simulink model "sudarshan_1"  (R2022b)
settings: Solver=ode4  StartTime=0.0  StopTime=5  FixedStep=0.0001  RelTol=1e-3
settings Model: Creator=year2  LastModifiedBy=year2

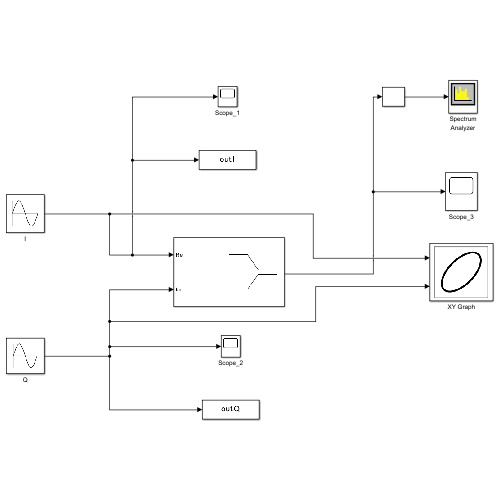
[thumbnail: Simulink's stored preview of the top-level diagram]
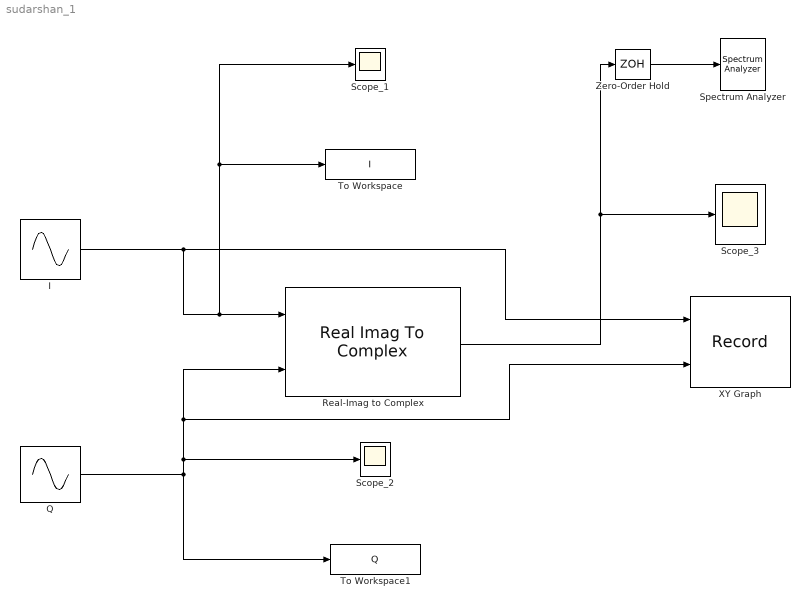
== system sudarshan_1 ==
  I : Sin  Frequency=100  Phase=pi/2  SampleTime=0
  Q : Sin  Frequency=100  SampleTime=0
  Real-Imag to Complex : RealImagToComplex
  Scope_1 : Scope
  Scope_2 : Scope
  Scope_3 : Scope
  Spectrum Analyzer : SpectrumAnalyzer
  To Workspace : ToWorkspace  VariableName=I  SaveFormat=Timeseries  SampleTime=-1
  To Workspace1 : ToWorkspace  VariableName=Q  SaveFormat=Timeseries  SampleTime=-1
  XY Graph : Record  FileSettingsInternal="{\"entries\":[{\"content\":{\"excelSettings\":{\"content\":{},\"type\":\"Streamout.ExcelSettings\"}},\"type\":\"Streamout.FileSettingStorage\",\"uuid\":\"9869a838-1e5d-41e2-a3ef-ea152b2475d8\"}],\"packageUris\":[\"http://schema.mathworks.com/mf0/streamout_blocks/R2020a\"],\"version\":\"1.0\"}"  Layout=[1 1]  SignalsInternal="{\"entries\":[{\"content\":{\"signals\":[{\"content\":{\"blockPath\":[\"sudarshan_1/XY Graph\"],\"channel\":[],\"dimensions\":[1],\"domain\":\"sudarshan_1/XY Graph\",\"lineColor\":\"#a2142f\",\"plots\":[1],\"port\":1,\"sid\":[\"\"],\"signalID\":933,\"signalName\":\"I\"},\"type\":\"RecordBlkView.Signal\",\"uuid\":\"0f210d62-b191-4474-a9fa-690a825850b4\"},{\"content\":{\"blockPath\":[\"sudarshan_1/XY Graph\"],\"channel\":[],\"dimensions\":[1],\"domain\":\"sudarshan_1/XY Graph\",\"lineColor\":\"#139fff\",\"plots\":[1],\"port\":2,\"sid\":[\"\"],\"signalID\":937,\"signalName\":\"Q\"},\"type\":\"RecordBlkView.Signal\",\"uuid\":\"0fb77e11-67ed-4f85-9229-98e8afdb45b5\"}]},\"type\":\"RecordBlkView.InputSignals\",\"uuid\":\"c6290ea5-0a28-4ce6-bd02-07c76cc485c4\"}],\"packageUris\":[\"http://schema.mathworks.com/mf0/streamout_blocks/R2020a\"],\"version\":\"1.0\"}"  VisualizationBindings="{\"xyplotplugin\":{\"info\":[{\"series\":[{\"bindingParametersList\":[{\"parameter\":\"X-Axis\",\"signalID\":933,\"signalName\":\"I\"},{\"parameter\":\"Y-Axis\",\"signalID\":937,\"signalName\":\"Q\"}],\"seriesID\":43396}],\"subplotID\":1}]}}"  CompatibilityTag=XY  st=-1
  Zero-Order Hold : ZeroOrderHold  SampleTime=-1
  wires:
  Q/1 -> To Workspace1/1, XY Graph/2, Real-Imag to Complex/2, Scope_2/1
  I/1 -> XY Graph/1, To Workspace/1, Scope_1/1, Real-Imag to Complex/1
  Real-Imag to Complex/1 -> Scope_3/1, Zero-Order Hold/1
  Zero-Order Hold/1 -> Spectrum Analyzer/1
